simulink model "main"  (R2024b)
settings: Solver=FixedStepAuto  StartTime=0.0  StopTime=10  FixedStep=Ts  RelTol=1e-3
values from neighbouring files (symbols this model uses):
  Frr = 1    [getItRunning.m]
  v0 = 10    [getItRunning.m]
libraries: cstblocks x1
settings Model: Creator=marti  LastModifiedBy=marti

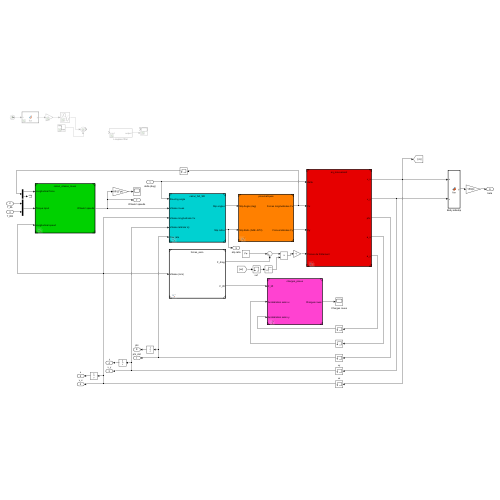
[thumbnail: Simulink's stored preview of the top-level diagram]
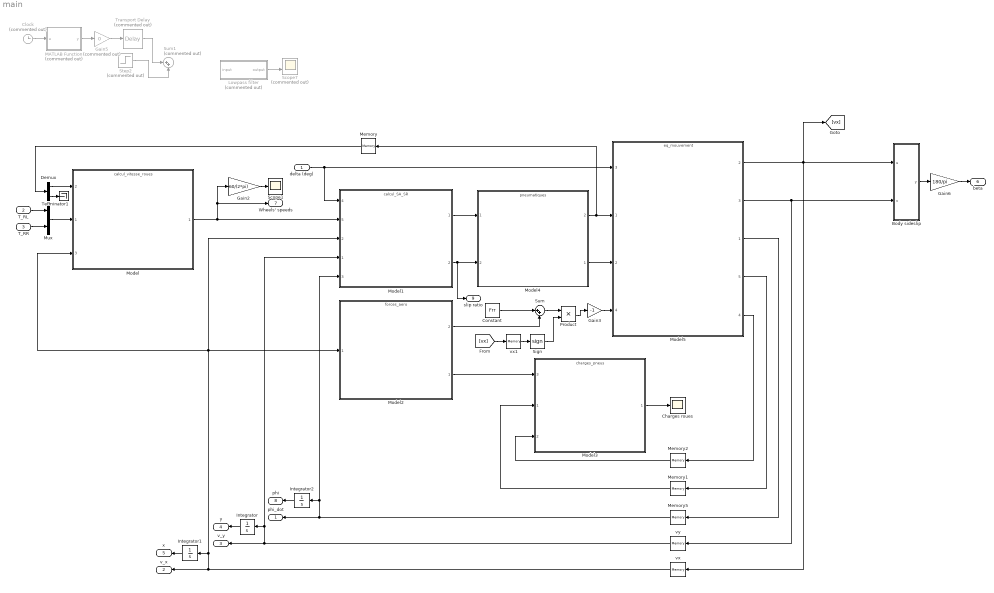
== system main ==
  delta (deg) : Inport
  T_RL : Inport  Port=2
  T_RR : Inport  Port=3
  Body sideslip : MATLAB Function  TreatAsAtomicUnit=on
  Charges roues : Scope
  Clock : Clock  Commented=on
  Constant : Constant  Value=Frr
  Demux : Demux  Outputs=2
  Gain2 : Gain  Gain=60/(2*pi)
  Gain3 : Gain  Gain=-1
  Gain5 : Gain  Commented=on  Gain=0
  Gain6 : Gain  Gain=180/pi
  Integrator : Integrator
  Integrator1 : Integrator
  Integrator2 : Integrator
  Lowpass filter : Subsystem  Commented=on
  MATLAB Function : MATLAB Function  Commented=on  TreatAsAtomicUnit=on
  Memory : Memory  InitialCondition=[0 0 0 0]
  Memory1 : Memory
  Memory2 : Memory
  Memory5 : Memory
  Model : ModelReference  ModelNameDialog=calcul_vitesse_roues.slx  SimulationMode=Normal  ModelReferenceVersion=1.21
      settings: PortSchema="{\"entries\":[{\"content\":{\"sides\":[{\"content\":{\"connectorIds\":[\"In2\",\"In1\",\"In3\"]},\"type\":\"ConnectorPlacement.EquallySpacedRectSide\",\"uuid\":\"32c61a1f-6c57-499a-b866-aceaf52d28d2\"},{\"content\":{\"connectorIds\":[\"Out1\"],\"side\":\"RIGHT\"},\"type\":\"ConnectorPlacement.EquallySpacedRectSide\",\"uuid\":\"cffac577-4d60-419d-9ad2-4916db655c57\"},{\"content\":{\"side\":\"TOP\"},\"type\":\"ConnectorPlacement.EquallySpacedRectSide\",\"uuid\":\"34bdae6d-bec4-41a0-a8ed-c228eaa34691\"}]},\"type\":\"ConnectorPlacement.EquallySpacedConnector\",\"uuid\":\"84af7d52-f463-465c-ba60-2639f593163f\"}],\"packageUris\":[\"http://schema.mathworks.com/mf0/Connector/R2020b\"],\"version\":\"1.0\"}"
  Model1 : ModelReference  ModelNameDialog=calcul_SA_SR.slx  SimulationMode=Normal  ModelReferenceVersion=1.25
      settings: PortSchema="{\"entries\":[{\"content\":{\"sides\":[{\"content\":{\"connectorIds\":[\"In4\",\"In5\",\"In2\",\"In1\",\"In3\"]},\"type\":\"ConnectorPlacement.EquallySpacedRectSide\",\"uuid\":\"04201970-b5ae-4970-bbc5-44410850cae5\"},{\"content\":{\"connectorIds\":[\"Out1\",\"Out2\"],\"side\":\"RIGHT\"},\"type\":\"ConnectorPlacement.EquallySpacedRectSide\",\"uuid\":\"ab4d4869-684a-4026-8884-27d4e324b480\"},{\"content\":{\"side\":\"TOP\"},\"type\":\"ConnectorPlacement.EquallySpacedRectSide\",\"uuid\":\"05423dc3-4c94-48e1-85fd-0de66489003e\"}]},\"type\":\"ConnectorPlacement.EquallySpacedConnector\",\"uuid\":\"2b086429-66dd-48fe-b956-28c27be60a2d\"}],\"packageUris\":[\"http://schema.mathworks.com/mf0/Connector/R2020b\"],\"version\":\"1.0\"}"
  Model2 : ModelReference  ModelNameDialog=forces_aero.slx  SimulationMode=Normal  ModelReferenceVersion=1.4
      settings: PortSchema="{\"entries\":[{\"content\":{\"sides\":[{\"content\":{\"connectorIds\":[\"In1\"]},\"type\":\"ConnectorPlacement.EquallySpacedRectSide\",\"uuid\":\"36e8b1bd-3fb4-4164-87a8-b8a924d0920e\"},{\"content\":{\"connectorIds\":[\"Out2\",\"Out1\"],\"side\":\"RIGHT\"},\"type\":\"ConnectorPlacement.EquallySpacedRectSide\",\"uuid\":\"44b00b7a-cae6-466b-a7ba-191ad477ad1a\"},{\"content\":{\"side\":\"TOP\"},\"type\":\"ConnectorPlacement.EquallySpacedRectSide\",\"uuid\":\"ce0b7025-a6f5-43b6-8b2e-4f7110b22b08\"}]},\"type\":\"ConnectorPlacement.EquallySpacedConnector\",\"uuid\":\"fa91ac53-771c-475b-9f30-77799fcbe46a\"}],\"packageUris\":[\"http://schema.mathworks.com/mf0/Connector/R2020b\"],\"version\":\"1.0\"}"
  Model3 : ModelReference  ModelNameDialog=charges_pneus.slx  SimulationMode=Normal  ModelReferenceVersion=1.18
      settings: PortSchema="{\"entries\":[{\"content\":{\"sides\":[{\"content\":{\"connectorIds\":[\"In3\",\"In1\",\"In2\"]},\"type\":\"ConnectorPlacement.EquallySpacedRectSide\",\"uuid\":\"32c61a1f-6c57-499a-b866-aceaf52d28d2\"},{\"content\":{\"connectorIds\":[\"Out1\"],\"side\":\"RIGHT\"},\"type\":\"ConnectorPlacement.EquallySpacedRectSide\",\"uuid\":\"cffac577-4d60-419d-9ad2-4916db655c57\"},{\"content\":{\"side\":\"TOP\"},\"type\":\"ConnectorPlacement.EquallySpacedRectSide\",\"uuid\":\"34bdae6d-bec4-41a0-a8ed-c228eaa34691\"}]},\"type\":\"ConnectorPlacement.EquallySpacedConnector\",\"uuid\":\"84af7d52-f463-465c-ba60-2639f593163f\"}],\"packageUris\":[\"http://schema.mathworks.com/mf0/Connector/R2020b\"],\"version\":\"1.0\"}"
  Model4 : ModelReference  ModelNameDialog=pneumatiques.slx  SimulationMode=Normal  ModelReferenceVersion=1.24
      settings: PortSchema="{\"entries\":[{\"content\":{\"sides\":[{\"content\":{\"connectorIds\":[\"In1\",\"In2\"]},\"type\":\"ConnectorPlacement.EquallySpacedRectSide\",\"uuid\":\"aa9afb45-c7cc-47c2-a353-b159ebe33fc0\"},{\"content\":{\"connectorIds\":[\"Out2\",\"Out1\"],\"side\":\"RIGHT\"},\"type\":\"ConnectorPlacement.EquallySpacedRectSide\",\"uuid\":\"99ac261d-830b-4c4d-b54d-d5870e19fd84\"},{\"content\":{\"side\":\"TOP\"},\"type\":\"ConnectorPlacement.EquallySpacedRectSide\",\"uuid\":\"130b3d1d-6b2b-41ab-b5a2-95b935e32e22\"}]},\"type\":\"ConnectorPlacement.EquallySpacedConnector\",\"uuid\":\"701cb8d3-48d4-40f6-b223-8d3552990209\"}],\"packageUris\":[\"http://schema.mathworks.com/mf0/Connector/R2020b\"],\"version\":\"1.0\"}"
  Model5 : ModelReference  ModelNameDialog=eq_mouvement.slx  SimulationMode=Normal  ModelReferenceVersion=1.16
      settings: PortSchema="{\"entries\":[{\"content\":{\"sides\":[{\"content\":{\"connectorIds\":[\"In3\",\"In1\",\"In2\",\"In4\"]},\"type\":\"ConnectorPlacement.EquallySpacedRectSide\",\"uuid\":\"7adc66df-ae88-4ff9-8d9d-989933ee26de\"},{\"content\":{\"connectorIds\":[\"Out2\",\"Out3\",\"Out1\",\"Out5\",\"Out4\"],\"side\":\"RIGHT\"},\"type\":\"ConnectorPlacement.EquallySpacedRectSide\",\"uuid\":\"fc5e31fc-1ddd-4d83-91f3-0c7f32150fd7\"},{\"content\":{\"side\":\"TOP\"},\"type\":\"ConnectorPlacement.EquallySpacedRectSide\",\"uuid\":\"7ddc969d-b7ab-4ed3-9e24-42b0de14a816\"}]},\"type\":\"ConnectorPlacement.EquallySpacedConnector\",\"uuid\":\"ce6a4464-9d25-4f4c-9109-1582c6857295\"}],\"packageUris\":[\"http://schema.mathworks.com/mf0/Connector/R2020b\"],\"version\":\"1.0\"}"
  Mux : Mux  Inputs=2
  Product : Product
  Scope1 : Scope
  Scope7 : Scope  Commented=on  NumInputPorts=2
  Sign : Signum
  Step2 : Step  Commented=on  Time=5  Before=10  After=-10  SampleTime=0
  Sum : Sum  Inputs=|++
  Sum1 : Sum  Commented=on  Inputs=|++
  Terminator1 : Terminator
  Transport Delay : TransportDelay  Commented=on  BufferSize=10240
  vx : Memory  InitialCondition=v0
  vx1 : Memory  InitialCondition=v0
  vy : Memory
  phi_dot : Outport
  v_x : Outport  Port=2
  v_y : Outport  Port=3
  y : Outport  Port=4
  x : Outport  Port=5
  beta : Outport  Port=6
  Wheels' speeds : Outport  Port=7
  phi : Outport  Port=8
  slip ratio : Outport  Port=9
  wires:
  Model2/1 -> Model3/3
  Model2/2 -> Sum/2
  Model/1 -> Model1/5, Gain2/1, Wheels' speeds/1
  Model5/1 -> Memory5/1
  Model5/3 -> vy/1, Body sideslip/2(v)
  Model5/4 -> Memory2/1
  Model5/5 -> Memory1/1
  Model5/2 -> [vx], vx/1, Body sideslip/1(u)
  Mux/1 -> Model/1
  Memory/1 -> Demux/1
  Demux/1 -> Model/2
  Demux/2 -> Terminator1/1
  Memory1/1 -> Model3/1
  Memory2/1 -> Model3/2
  vy/1 -> Model1/1, Integrator/1, v_y/1
  vx/1 -> Model1/2, Model/3, Model2/1, Integrator1/1, v_x/1
  Memory5/1 -> Model1/3, Integrator2/1, phi_dot/1
  Model3/1 -> Charges roues/1
  Model1/1 -> Model4/1
  Gain2/1 -> Scope1/1
  T_RL/1 -> Mux/1
  T_RR/1 -> Mux/2
  Model1/2 -> slip ratio/1, Model4/2
  Constant/1 -> Sum/1
  Gain3/1 -> Model5/4
  Model4/1 -> Model5/2
  Integrator/1 -> y/1
  Integrator1/1 -> x/1
  Integrator2/1 -> phi/1
  Model4/2 -> Model5/1, Memory/1
  Body sideslip/1(y) -> Gain6/1
  Gain6/1 -> beta/1
  Gain5/1 -> Transport Delay/1
  Clock/1 -> MATLAB Function/1(u)
  Step2/1 -> Sum1/2
  Transport Delay/1 -> Sum1/1
  MATLAB Function/1(y) -> Gain5/1
  delta (deg)/1 -> Model1/4, Model5/3
  Lowpass filter/1(output) -> Scope7/2
  [vx] -> vx1/1
  Sum/1 -> Product/1
  Product/1 -> Gain3/1
  Sign/1 -> Product/2
  vx1/1 -> Sign/1

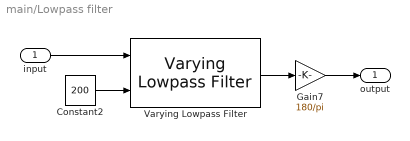
== system main/Lowpass filter ==
  input : Inport
  Constant2 : Constant  Value=200
  Gain7 : Gain  Gain=180/pi
  Varying Lowpass Filter : cstblocks/Linear Parameter Varying/Varying Lowpass Filter  N=1
  output : Outport
  wires:
  Constant2/1 -> Varying Lowpass Filter/2
  Varying Lowpass Filter/1 -> Gain7/1
  input/1 -> Varying Lowpass Filter/1
  Gain7/1 -> output/1

== matlab function main/MATLAB Function ==
  data: u input; y output
function y = fcn(u)
   y = 1 - exp(-u/2);
end

== matlab function main/Body sideslip ==
  data: u input; y output; v input
function y = fcn(u,v)

y = atan(v/u);
end
